simulink model "double_loop_counters"  (R2017b)
settings: Solver=FixedStepDiscrete  StartTime=0.0  StopTime=1  FixedStep=0.005  RelTol=1e-3  EnableMultiTasking=on
settings Model: Creator=Parker  LastModifiedBy=pthb3
settings SolverCC: AlgebraicLoopSolver=LineSearch  PositivePriorityOrder=on  AutoInsertRateTranBlk=on  InsertRTBMode=Always
settings CodeAppCC: StateflowObjectComments=on

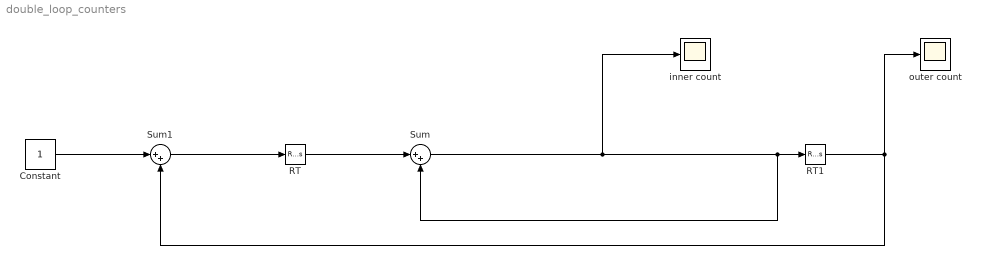
== system double_loop_counters ==
  Constant : Constant
  RT : RateTransition  OutPortSampleTime=0.005
  RT1 : RateTransition  OutPortSampleTime=0.05
  Sum : Sum  Inputs=|++
  Sum1 : Sum  Inputs=|++
  inner count : Scope
  outer count : Scope
  wires:
  Sum/1 -> inner count/1, Sum/2, RT1/1
  RT1/1 -> Sum1/2, outer count/1
  Sum1/1 -> RT/1
  Constant/1 -> Sum1/1
  RT/1 -> Sum/1
